simulink model "system2"  (R2018b)
settings: Solver=ode1  StartTime=0.0  StopTime=10  FixedStep=.001  RelTol=1e-3
values from neighbouring files (symbols this model uses):
  A3 = [0  1  0; 0  0  1; 4374  -81  -36]    [matlab.mat]
  B3 = [0 0 1]    [matlab.mat]
  C3 = [39.6 4 0]    [matlab.mat]
  C3B = [1 0 0]    [matlab.mat]
  K3 = [4380 -70 -30]    [matlab.mat]
  K3B = [4380 -70 -30]    [matlab.mat]
  L3 = [0.25002206018 -3.22521839578 129.179662118]    [matlab.mat]
libraries: cstblocks x1
settings Model: Creator=Abraham Pérez  LastModifiedBy=Abraham Pérez
settings SolverCC: InitialStep=.001

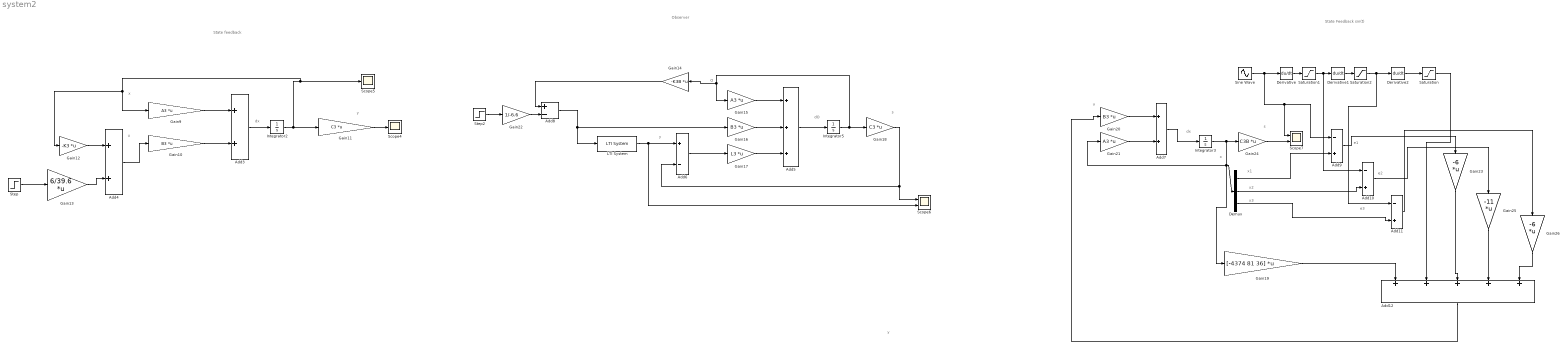
== system system2 ==
  note: e3
  note: e2
  note: e1
  note: x3
  note: x2
  note: x1
  note: x
  note: u
  note: State feedback
  note: dx
  note: x
  note: y
  note: u
  note: Observer
  note: dO
  note: y
  note: s
  note: y
  note: O
  note: s
  note: dx
  note: State Feedback sin(t)
  Add10 : Sum  Inputs=-+
  Add11 : Sum  Inputs=-+
  Add12 : Sum  Inputs=+++++
  Add3 : Sum
  Add4 : Sum
  Add5 : Sum  Inputs=+++
  Add6 : Sum  Inputs=+-
  Add7 : Sum
  Add8 : Sum  Inputs=+-
  Add9 : Sum  Inputs=-+
  Demux : Demux  Outputs=3
  Derivative : Derivative
  Derivative1 : Derivative
  Derivative2 : Derivative
  Gain10 : Gain  Gain=B3  Multiplication=Matrix(K*u)
  Gain11 : Gain  Gain=C3  Multiplication=Matrix(K*u)
  Gain12 : Gain  Gain=-K3  Multiplication=Matrix(K*u)
  Gain13 : Gain  Gain=6/39.6  Multiplication=Matrix(K*u)
  Gain14 : Gain  Gain=-K3B  Multiplication=Matrix(K*u)
  Gain15 : Gain  Gain=A3  Multiplication=Matrix(K*u)
  Gain16 : Gain  Gain=B3  Multiplication=Matrix(K*u)
  Gain17 : Gain  Gain=L3  Multiplication=Matrix(K*u)
  Gain18 : Gain  Gain=C3  Multiplication=Matrix(K*u)
  Gain19 : Gain  Gain=[-4374 81 36]  Multiplication=Matrix(K*u)
  Gain20 : Gain  Gain=B3  Multiplication=Matrix(K*u)
  Gain21 : Gain  Gain=A3  Multiplication=Matrix(K*u)
  Gain22 : Gain  Gain=1/-6.6
  Gain23 : Gain  Gain=-6  Multiplication=Matrix(K*u)
  Gain24 : Gain  Gain=C3B  Multiplication=Matrix(K*u)
  Gain25 : Gain  Gain=-11  Multiplication=Matrix(K*u)
  Gain26 : Gain  Gain=-6  Multiplication=Matrix(K*u)
  Gain9 : Gain  Gain=A3  Multiplication=Matrix(K*u)
  Integrator2 : Integrator  InitialCondition=[-1 .5 .5 ]
  Integrator3 : Integrator  InitialCondition=[1 0 -1]
  Integrator5 : Integrator  InitialCondition=[1 0 -1]
  LTI System : cstblocks/LTI System  sys=G3  IC=[]
  Saturation : Saturate  UpperLimit=1  LowerLimit=-1
  Saturation1 : Saturate  UpperLimit=1  LowerLimit=-1
  Saturation2 : Saturate  UpperLimit=1  LowerLimit=-1
  Scope4 : Scope
  Scope5 : Scope
  Scope6 : Scope  NumInputPorts=2
  Scope7 : Scope  NumInputPorts=2
  Sine Wave : Sin  Amplitude=.05  SampleTime=0
  Step : Step  After=26  SampleTime=0
  Step2 : Step  After=52  SampleTime=0
  wires:
  Step/1 -> Gain13/1
  Gain12/1 -> Add4/1
  Gain13/1 -> Add4/2
  Add4/1 -> Gain10/1
  Gain10/1 -> Add3/2
  Gain11/1 -> Scope4/1
  Gain9/1 -> Add3/1
  Add3/1 -> Integrator2/1
  Integrator2/1 -> Gain11/1, Scope5/1, Gain9/1, Gain12/1
  Gain17/1 -> Add5/3
  LTI System/1 -> Scope6/2, Add6/1
  Add6/1 -> Gain17/1
  Integrator5/1 -> Gain18/1, Gain15/1, Gain14/1
  Add5/1 -> Integrator5/1
  Gain15/1 -> Add5/1
  Gain16/1 -> Add5/2
  Gain14/1 -> Add8/1
  Gain22/1 -> Add8/2
  Step2/1 -> Gain22/1
  Add8/1 -> Gain16/1, LTI System/1
  Gain18/1 -> Scope6/1, Add6/2
  Gain20/1 -> Add7/1
  Add7/1 -> Integrator3/1
  Gain21/1 -> Add7/2
  Derivative1/1 -> Saturation2/1
  Demux/1 -> Add9/2
  Demux/2 -> Add10/2
  Demux/3 -> Add11/2
  Integrator3/1 -> Gain19/1, Gain21/1, Demux/1, Gain24/1
  Gain19/1 -> Add12/1
  Add9/1 -> Gain23/1
  Gain23/1 -> Add12/3
  Add10/1 -> Gain25/1
  Gain25/1 -> Add12/4
  Add11/1 -> Gain26/1
  Gain26/1 -> Add12/5
  Add12/1 -> Gain20/1
  Derivative2/1 -> Saturation/1
  Saturation2/1 -> Add11/1, Derivative2/1
  Saturation/1 -> Add12/2
  Gain24/1 -> Scope7/2
  Saturation1/1 -> Add10/1, Derivative1/1
  Derivative/1 -> Saturation1/1
  Sine Wave/1 -> Scope7/1, Add9/1, Derivative/1
